simulink model "Simulink"  (R2024b)
settings: Solver=VariableStepAuto  StartTime=0.0  StopTime=100  RelTol=1e-3
values from neighbouring files (symbols this model uses):
  btm = 2.348e-9    (= 2.348e-09)    [MATLABCode.m]
  Jm = 172e-6    (= 0.000172)    [MATLABCode.m]
  kd = 1e-100    [MATLABCode.m]
  ki = 0    [MATLABCode.m]
  kp = 1    [MATLABCode.m]
  Ktm = 20.2e-3    (= 0.0202)    [MATLABCode.m]
  Kv = 0.0202    [MATLABCode.m]
  Lm = 860e-6    (= 0.00086)    [MATLABCode.m]
  R = 8    [MATLABCode.m]
libraries: slpidlib x2
settings Model: Creator=mwali  LastModifiedBy=user
settings RTWCC: GPUComputeCapability=3.5

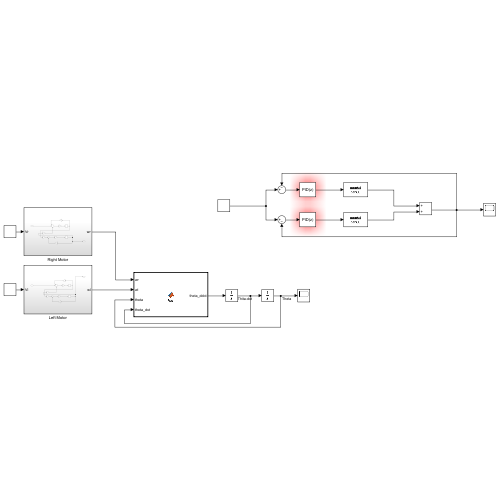
[thumbnail: Simulink's stored preview of the top-level diagram]
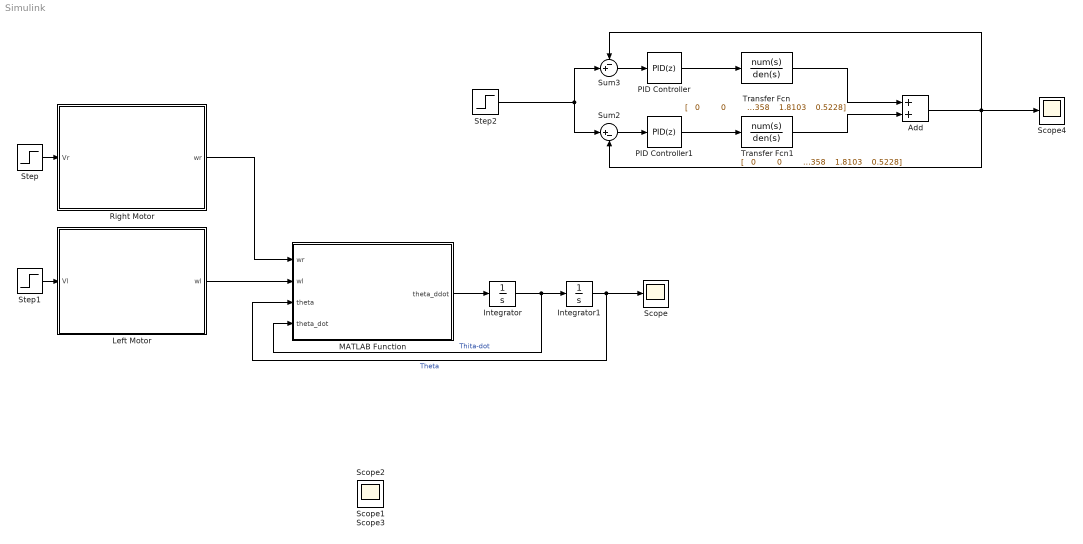
== system Simulink ==
  Add : Sum
  Integrator : Integrator
  Integrator1 : Integrator
  Left Motor : Subsystem
  MATLAB Function : MATLAB Function  TreatAsAtomicUnit=on
  PID Controller : slpidlib/PID Controller  Controller=PID  Form=Parallel  TimeDomain=Discrete-time  UseExternalTs=off  SampleTime=-1  IntegratorMethod=Forward Euler  FilterMethod=Forward Euler  ControllerParametersSource=internal  P=kp  I=ki  UseKiTs=off  D=kd  UseExternalDerivativeSource=off  N=100  UseFilter=on  TunerSelectOption=Transfer Function Based (PID Tuner App)  InitialConditionSource=internal  InitialConditionForIntegrator=0  InitialConditionForFilter=0  DifferentiatorICPrevScaledInput=0  ExternalReset=none  TrackingMode=off  Kt=1  LimitOutput=off  SatLimitsSource=internal  UpperSaturationLimit=inf  LowerSaturationLimit=-inf  LinearizeAsGain=on  AntiWindupMode=none  Kb=1  LimitIntegrator=off  UpperIntegratorSaturationLimit=inf  LowerIntegratorSaturationLimit=-inf  POutMin=[]  POutMax=[]  IOutMin=[]  IOutMax=[]  DOutMin=[]  DOutMax=[]  NOutMin=[]  NOutMax=[]  SumOutMin=[]  SumOutMax=[]  SaturationOutMin=[]  SaturationOutMax=[]  PParamMin=[]  PParamMax=[]  IParamMin=[]  IParamMax=[]  DParamMin=[]  DParamMax=[]  NParamMin=[]  NParamMax=[]  KbParamMin=[]  KbParamMax=[]  KtParamMin=[]  KtParamMax=[]  KbOutMin=[]  KbOutMax=[]  KtOutMin=[]  KtOutMax=[]  IntegratorOutMin=[]  IntegratorOutMax=[]  FilterOutMin=[]  FilterOutMax=[]  SumI1OutMin=[]  SumI1OutMax=[]  SumI2OutMin=[]  SumI2OutMax=[]  SumI3OutMin=[]  SumI3OutMax=[]  SumI4OutMin=[]  SumI4OutMax=[]  SumDOutMin=[]  SumDOutMax=[]  DifferentiatorOutMin=[]  DifferentiatorOutMax=[]  FilterDiffOutCoefMin=[]  FilterDiffOutCoefMax=[]  ReciprocalOutMin=[]  ReciprocalOutMax=[]  SumDenOutMin=[]  SumDenOutMax=[]  SumNumOutMin=[]  SumNumOutMax=[]  DivideOutMin=[]  DivideOutMax=[]  UdiffTsProdOutMin=[]  UdiffTsProdOutMax=[]  NTsProdOutMin=[]  NTsProdOutMax=[]  UintegralTsProdOutMin=[]  UintegralTsProdOutMax=[]  UngainTsProdOutMin=[]  UngainTsProdOutMax=[]  ClampingZeroOutDataTypeStr=Inherit: Inherit via back propagation  ClampingZeroOutMin=[]  ClampingZeroOutMax=[]  FilterDenConstantOutDataTypeStr=Inherit: Inherit via back propagation  FilterDenConstantOutMin=[]  FilterDenConstantOutMax=[]  PCopyOutDataTypeStr=Inherit: Inherit via back propagation  PCopyOutMin=[]  PCopyOutMax=[]  NCopyOutDataTypeStr=Inherit: Inherit via back propagation  NCopyOutMin=[]  NCopyOutMax=[]  IntegratorContinuousStateAttributes=''  IntegratorStateMustResolveToSignalObject=off  IntegratorRTWStateStorageClass=Auto  FilterContinuousStateAttributes=''  FilterStateMustResolveToSignalObject=off  FilterRTWStateStorageClass=Auto  ParallelPVariant=InternalParameters  IdealPVariant=Disabled  IVariant=InternalParameters  DVariant=InternalParameters  IntegratorVariant=Discrete  SatVariant=Disabled  AWVariant=Passthrough  PCopyVariant=Disabled  TRVariant=Disabled  FdbkBlocksVariant=Forward  IdealPFdbkVariant=Disabled  SatFdbkVariant=Disabled  DerivativeFilterVariant=ForwardEulerFilter  NVariant=InternalParameters  NCopyVariant=Disabled  FilterICVariant=InternalICsFilter  IntegratorICVariant=InternalICs  ExternalResetVariant=Disabled  TRSumVariant=Passthrough  SumFdbkVariant=Disabled  SumVariant=Sum_PID  TsampFilterVariant=InternalTs  TsampNgainVariant=Passthrough  TsampIntegralVariant=Disabled_SignalSpec  ExternalSaturationOutDataTypeStr=Inherit: Same as second input  DerivativeSourceVariant=ErrorSignal  PreIntVariant=InternalPreInt
  PID Controller1 : slpidlib/PID Controller  Controller=PID  Form=Parallel  TimeDomain=Discrete-time  UseExternalTs=off  SampleTime=-1  IntegratorMethod=Forward Euler  FilterMethod=Forward Euler  ControllerParametersSource=internal  P=kp  I=ki  UseKiTs=off  D=kd  UseExternalDerivativeSource=off  N=100  UseFilter=on  TunerSelectOption=Transfer Function Based (PID Tuner App)  InitialConditionSource=internal  InitialConditionForIntegrator=0  InitialConditionForFilter=0  DifferentiatorICPrevScaledInput=0  ExternalReset=none  TrackingMode=off  Kt=1  LimitOutput=off  SatLimitsSource=internal  UpperSaturationLimit=inf  LowerSaturationLimit=-inf  LinearizeAsGain=on  AntiWindupMode=none  Kb=1  LimitIntegrator=off  UpperIntegratorSaturationLimit=inf  LowerIntegratorSaturationLimit=-inf  POutMin=[]  POutMax=[]  IOutMin=[]  IOutMax=[]  DOutMin=[]  DOutMax=[]  NOutMin=[]  NOutMax=[]  SumOutMin=[]  SumOutMax=[]  SaturationOutMin=[]  SaturationOutMax=[]  PParamMin=[]  PParamMax=[]  IParamMin=[]  IParamMax=[]  DParamMin=[]  DParamMax=[]  NParamMin=[]  NParamMax=[]  KbParamMin=[]  KbParamMax=[]  KtParamMin=[]  KtParamMax=[]  KbOutMin=[]  KbOutMax=[]  KtOutMin=[]  KtOutMax=[]  IntegratorOutMin=[]  IntegratorOutMax=[]  FilterOutMin=[]  FilterOutMax=[]  SumI1OutMin=[]  SumI1OutMax=[]  SumI2OutMin=[]  SumI2OutMax=[]  SumI3OutMin=[]  SumI3OutMax=[]  SumI4OutMin=[]  SumI4OutMax=[]  SumDOutMin=[]  SumDOutMax=[]  DifferentiatorOutMin=[]  DifferentiatorOutMax=[]  FilterDiffOutCoefMin=[]  FilterDiffOutCoefMax=[]  ReciprocalOutMin=[]  ReciprocalOutMax=[]  SumDenOutMin=[]  SumDenOutMax=[]  SumNumOutMin=[]  SumNumOutMax=[]  DivideOutMin=[]  DivideOutMax=[]  UdiffTsProdOutMin=[]  UdiffTsProdOutMax=[]  NTsProdOutMin=[]  NTsProdOutMax=[]  UintegralTsProdOutMin=[]  UintegralTsProdOutMax=[]  UngainTsProdOutMin=[]  UngainTsProdOutMax=[]  ClampingZeroOutDataTypeStr=Inherit: Inherit via back propagation  ClampingZeroOutMin=[]  ClampingZeroOutMax=[]  FilterDenConstantOutDataTypeStr=Inherit: Inherit via back propagation  FilterDenConstantOutMin=[]  FilterDenConstantOutMax=[]  PCopyOutDataTypeStr=Inherit: Inherit via back propagation  PCopyOutMin=[]  PCopyOutMax=[]  NCopyOutDataTypeStr=Inherit: Inherit via back propagation  NCopyOutMin=[]  NCopyOutMax=[]  IntegratorContinuousStateAttributes=''  IntegratorStateMustResolveToSignalObject=off  IntegratorRTWStateStorageClass=Auto  FilterContinuousStateAttributes=''  FilterStateMustResolveToSignalObject=off  FilterRTWStateStorageClass=Auto  ParallelPVariant=InternalParameters  IdealPVariant=Disabled  IVariant=InternalParameters  DVariant=InternalParameters  IntegratorVariant=Discrete  SatVariant=Disabled  AWVariant=Passthrough  PCopyVariant=Disabled  TRVariant=Disabled  FdbkBlocksVariant=Forward  IdealPFdbkVariant=Disabled  SatFdbkVariant=Disabled  DerivativeFilterVariant=ForwardEulerFilter  NVariant=InternalParameters  NCopyVariant=Disabled  FilterICVariant=InternalICsFilter  IntegratorICVariant=InternalICs  ExternalResetVariant=Disabled  TRSumVariant=Passthrough  SumFdbkVariant=Disabled  SumVariant=Sum_PID  TsampFilterVariant=InternalTs  TsampNgainVariant=Passthrough  TsampIntegralVariant=Disabled_SignalSpec  ExternalSaturationOutDataTypeStr=Inherit: Same as second input  DerivativeSourceVariant=ErrorSignal  PreIntVariant=InternalPreInt
  Right Motor : Subsystem
  Scope{,1..4} (5 alike) : Scope
  Step : Step  SampleTime=0
  Step1 : Step  SampleTime=0
  Step2 : Step  After=0.001  SampleTime=0
  Sum2 : Sum  Inputs=|+-
  Sum3 : Sum  Inputs=-+|
  Transfer Fcn : TransferFcn  Numerator="[   0         0         0   - -5.531e-06 -562.7937]"  Denominator="1.0e+04 *[ 0.0001    0.9302    0.4358    1.8103    0.5228]"
  Transfer Fcn1 : TransferFcn  Numerator="[   0         0         0   5.531e-06 562.7937]"  Denominator="1.0e+04 *[ 0.0001    0.9302    0.4358    1.8103    0.5228]"
  wires:
  MATLAB Function/1(theta_ddot) -> Integrator/1
  Integrator/1 -> MATLAB Function/4(theta_dot), Integrator1/1  "Thita-dot"
  Integrator1/1 -> MATLAB Function/3(theta), Scope/1  "Theta"
  Right Motor/1(wr) -> MATLAB Function/1(wr)
  Left Motor/1(wl) -> MATLAB Function/2(wl)
  Step1/1 -> Left Motor/1(Vl)
  Step/1 -> Right Motor/1(Vr)
  Transfer Fcn/1 -> Add/1
  Sum2/1 -> PID Controller1/1
  PID Controller/1 -> Transfer Fcn/1
  Transfer Fcn1/1 -> Add/2
  PID Controller1/1 -> Transfer Fcn1/1
  Add/1 -> Sum3/1, Sum2/2, Scope4/1
  Step2/1 -> Sum3/2, Sum2/1
  Sum3/1 -> PID Controller/1

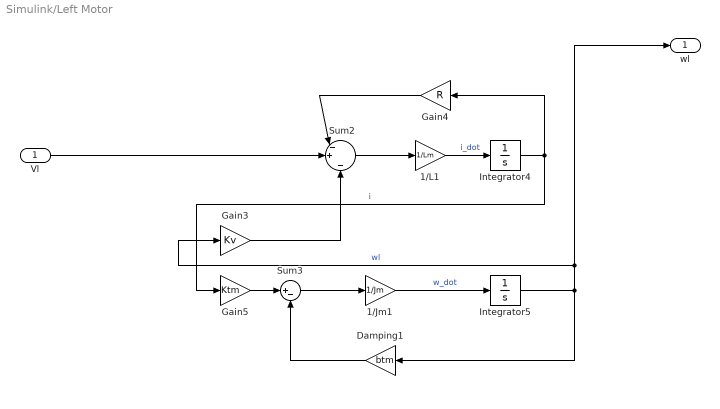
== system Simulink/Left Motor ==
  Vl : Inport
  1/Jm1 : Gain  Gain=1/Jm
  1/L1 : Gain  Gain=1/Lm
  Damping1 : Gain  Gain=btm
  Gain3 : Gain  Gain=Kv
  Gain4 : Gain  Gain=R
  Gain5 : Gain  Gain=Ktm
  Integrator4 : Integrator
  Integrator5 : Integrator
  Sum2 : Sum  Inputs=|-+|-
  Sum3 : Sum  Inputs=|+-
  wl : Outport
  wires:
  Integrator5/1 -> wl/1, Gain3/1, Damping1/1  "wl"
  Sum3/1 -> 1/Jm1/1
  1/L1/1 -> Integrator4/1  "i_dot"
  Damping1/1 -> Sum3/2
  Sum2/1 -> 1/L1/1
  Gain3/1 -> Sum2/3
  1/Jm1/1 -> Integrator5/1  "w_dot"
  Gain5/1 -> Sum3/1
  Integrator4/1 -> Gain5/1, Gain4/1  "i"
  Gain4/1 -> Sum2/1
  Vl/1 -> Sum2/2

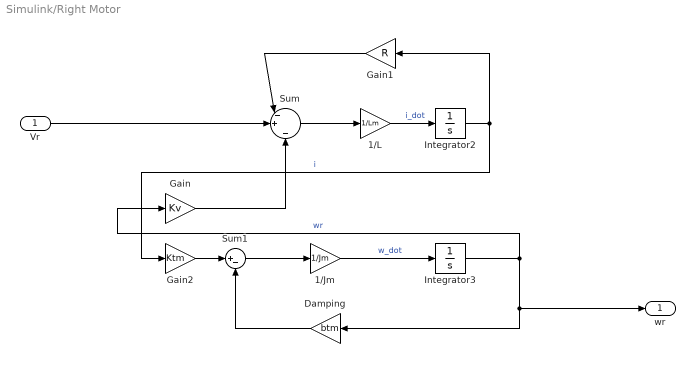
== system Simulink/Right Motor ==
  Vr : Inport
  1/Jm : Gain  Gain=1/Jm
  1/L : Gain  Gain=1/Lm
  Damping : Gain  Gain=btm
  Gain : Gain  Gain=Kv
  Gain1 : Gain  Gain=R
  Gain2 : Gain  Gain=Ktm
  Integrator2 : Integrator
  Integrator3 : Integrator
  Sum : Sum  Inputs=|-+|-
  Sum1 : Sum  Inputs=|+-
  wr : Outport
  wires:
  Gain/1 -> Sum/3
  1/L/1 -> Integrator2/1  "i_dot"
  Sum/1 -> 1/L/1
  Gain1/1 -> Sum/1
  Sum1/1 -> 1/Jm/1
  Damping/1 -> Sum1/2
  Gain2/1 -> Sum1/1
  Integrator3/1 -> Gain/1, wr/1, Damping/1  "wr"
  Integrator2/1 -> Gain2/1, Gain1/1  "i"
  1/Jm/1 -> Integrator3/1  "w_dot"
  Vr/1 -> Sum/2

== matlab function Simulink/MATLAB Function ==
  data: wr input; theta_ddot output; wl input; theta input; theta_dot input
function theta_ddot  = fcn(wr,wl,theta,theta_dot)
   
  L= 600e-3;
  Kt = 100e-6;
  Wo  = 2.0;        
  Lb = 300e-3;
  mb = 75e-3;
  g   = 9.81;
  J = 58.23e-3;
  bt = 10e-3;


    theta_ddot = ((2*L*Kt*Wo * (wr - wl)) - (bt * theta_dot) - ((Lb/2) * mb * g *  theta)) / J;
end
